simulink model "luenbrg_control_pole_placement"  (R2022b)
settings: Solver=VariableStepAuto  StartTime=0.0  StopTime=100  RelTol=1e-3
values from neighbouring files (symbols this model uses):
  A = [0 1; 0 -1/Tau]    [MPCsys_obs.m]    (also in derivative_control_LQ.m = [0 1; 0 -1/tau]; derivative_control_pole_placement.m = [0 1; 0 -1/tau])
  Aobs = A-L*C    [MPCsys_obs.m]    (also in derivative_control_LQ.m; derivative_control_pole_placement.m; luemberger_control_pole_placement.m)
  B = [0 K/Tau]'    [MPCsys_obs.m]    (also in derivative_control_LQ.m = [0 K/tau]'; derivative_control_pole_placement.m = [0 K/tau]')
  Bobs = [B, L]    [MPCsys_obs.m]    (also in derivative_control_LQ.m; derivative_control_pole_placement.m; luemberger_control_pole_placement.m)
  C = [1 0]    [MPCsys_obs.m]    (also in derivative_control_LQ.m; derivative_control_pole_placement.m)
  Cobs = eye(2)    [MPCsys_obs.m]    (also in derivative_control_LQ.m; derivative_control_pole_placement.m; luemberger_control_pole_placement.m)
  D = 0    [MPCsys_obs.m]    (also in derivative_control_LQ.m; derivative_control_pole_placement.m)
  Dobs = zeros(2, 2)    [MPCsys_obs.m]    (also in derivative_control_LQ.m; derivative_control_pole_placement.m; luemberger_control_pole_placement.m)
  K_v = K_eng(:, n+1:end)    [derivative_control_pole_placement.m]    (also in luemberger_control_pole_placement.m)
  K_x = K_eng(:, 1:n)    [derivative_control_pole_placement.m]    (also in luemberger_control_pole_placement.m)
settings Model: Creator=Davvy  LastModifiedBy=Davvy

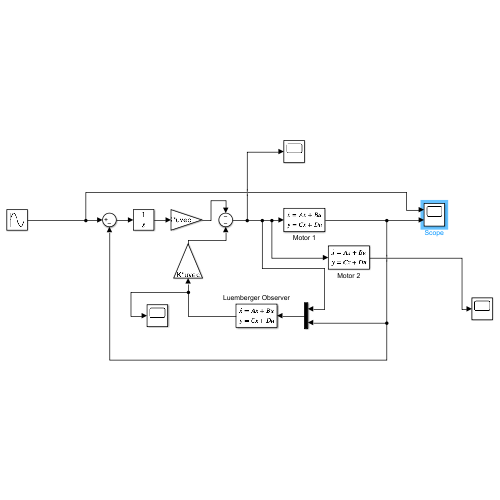
[thumbnail: Simulink's stored preview of the top-level diagram]
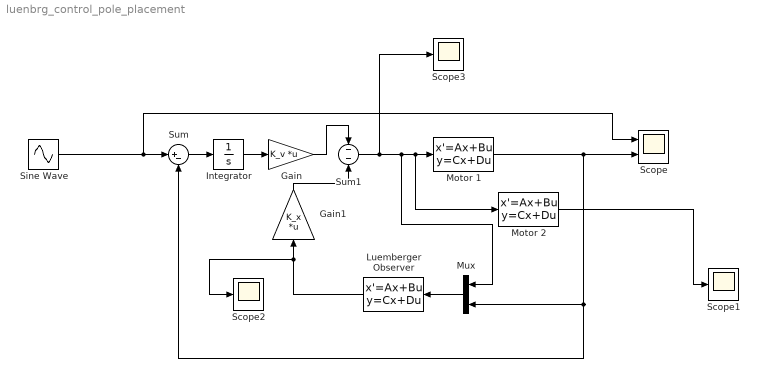
== system luenbrg_control_pole_placement ==
  Gain : Gain  Gain=K_v  Multiplication=Matrix(K*u) (u vector)
  Gain1 : Gain  Gain=K_x  Multiplication=Matrix(K*u) (u vector)
  Integrator : Integrator
  Luemberger Observer : StateSpace  A=Aobs  B=Bobs  C=Cobs  D=Dobs  InitialCondition=0
  Motor 1 : StateSpace  A=A  B=B  C=C  D=D  InitialCondition=0
  Motor 2 : StateSpace  A=A  B=B  C=eye(2)  D=[0;0]  InitialCondition=0
  Mux : Mux  Inputs=2
  Scope : Scope  NumInputPorts=2
  Scope1 : Scope
  Scope2 : Scope
  Scope3 : Scope
  Sine Wave : Sin  Frequency=60  SampleTime=0
  Sum : Sum  Inputs=|+-
  Sum1 : Sum  Inputs=--
  wires:
  Sine Wave/1 -> Scope/1, Sum/1
  Luemberger Observer/1 -> Scope2/1, Gain1/1
  Mux/1 -> Luemberger Observer/1
  Gain1/1 -> Sum1/2
  Sum1/1 -> Scope3/1, Mux/1, Motor 2/1, Motor 1/1
  Motor 1/1 -> Sum/2, Mux/2, Scope/2
  Gain/1 -> Sum1/1
  Sum/1 -> Integrator/1
  Integrator/1 -> Gain/1
  Motor 2/1 -> Scope1/1
